simulink model "immd_eff1"  (R2013a)
settings: Solver=ode4  StartTime=0.0  StopTime=0.5  FixedStep=Ts  RelTol=1e-3
values from neighbouring files (symbols this model uses):
  Cdc = 200e-6    (= 0.0002)    [immd_design_elen.m]    (also in immd_efficiency.m = 5e-05; immd_simulation_base.m = 5e-05; sixth_harmonic_report.m = 0.003)
  fout = 50    [immd_base_varyingmod.m]    (also in immd_design_elen.m; immd_efficiency.m; immd_simulation_base.m)
  Lload = Xload/wout_fund    [acemp_sixth.m]    (also in immd_base_varyingmod.m = Xload/wout; immd_design_elen.m = Xload/wout; immd_efficiency.m = Xload/wout; immd_simulation_base.m = Xload/wout)
  ma = 1    [IMMD_design_tool_v01.m]    (also in IMMD_design_tool_v02.m = 0.9; immd_base_varyingmod.m; immd_design_elen.m = 0.8; immd_efficiency.m = 0.85)
  phase = zeros(1,max_number_module)    [immd_base_varyingmod.m]    (also in immd_design_elen.m = [0 0 0 0]; immd_simulation_base.m = zeros(1,n))
  R1 = 5    [immd_efficiency.m]    (also in immd_simulation_base.m)
  Rload = Zload*pf    [acemp_sixth.m]    (also in immd_base_varyingmod.m; immd_design_elen.m; immd_efficiency.m; immd_simulation_base.m)
  Ts = 1e-6    (= 1e-06)    [acemp_sixth.m]    (also in immd_base_varyingmod.m = 1e-05; immd_design_elen.m; immd_efficiency.m; immd_simulation_base.m)
  V1 = Vdc*(R1+Rrefl)/Rrefl    (= 526.262626263)    [immd_efficiency.m]    (also in immd_simulation_base.m = 425.252525253)
  wout = 2*pi*fout    (= 314.159265359)    [immd_base_varyingmod.m]    (also in immd_design_elen.m; immd_efficiency.m; immd_simulation_base.m)
libraries: powerlib x21, powerlib_meascontrol x7
settings Model: Creator=ugurm  LastModifiedBy=ugurm

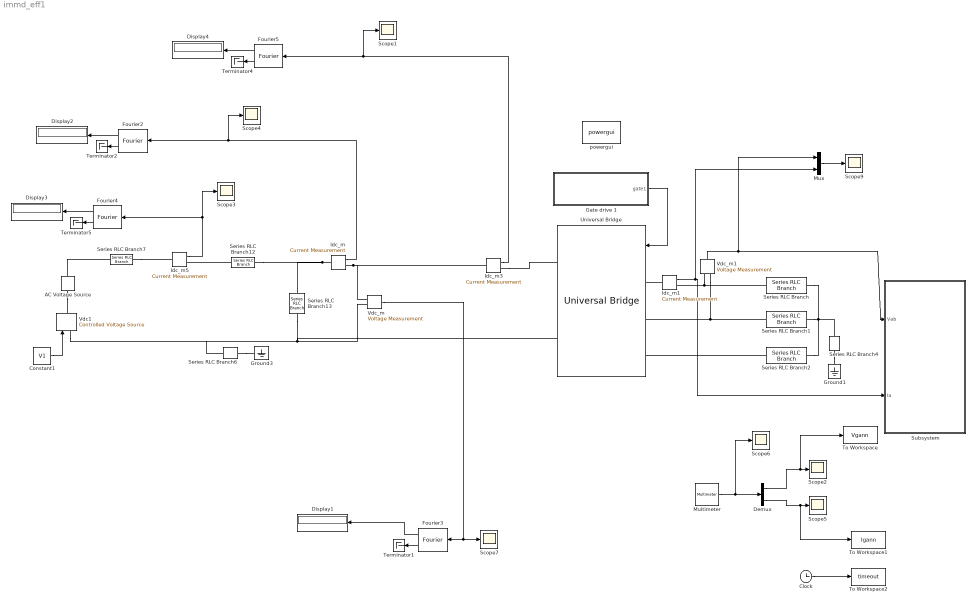
== system immd_eff1 ==
  AC Voltage Source : powerlib/Electrical Sources/AC Voltage Source  Amplitude=25  Phase=0  Frequency=6*fout  SampleTime=0  Measurements=None
  Clock : Clock
  Constant1 : Constant  Value=V1
  Demux : Demux  Outputs=2
  Display{1..4} (4 alike) : Display
  Fourier{2..5} (4 alike) : powerlib_meascontrol/Measurements/Fourier  Freq=fout  n=0  InInit=[0, 0]  Ts=Ts
  Gate drive 1 : Subsystem
  Ground1 : powerlib/Elements/Ground  LConnTagsString=a
  Ground3 : powerlib/Elements/Ground  LConnTagsString=a
  Idc_m{,1,3,5} (4 alike) : powerlib/Measurements/Current Measurement  PhasorSimulation=off  OutputType=Complex  PSBequivalent=0
  Multimeter : powerlib/Measurements/Multimeter  PhasorSimulation=off  OutputType=Complex  sel=[1 11]  L=16  Gain=[1 1]  yselected={'Usw1: Universal Bridge','Isw1: Universal Bridge'};  PSBOutputType=1  PSBequivalent=0  AxesSetting=[0,0.1,-100,100]  Display=0  SavedBlockNames=-11
  Mux : Mux  Inputs=2
  Scope{1..7,9} (8 alike) : Scope
      Scope1 settings: YMin=500  YMax=800  SaveName=idc1
      Scope2 settings: YMin=0  YMax=500
      Scope3 settings: YMin=24.9625  YMax=24.995  SaveName=ScopeData5
      Scope4 settings: YMin=500  YMax=800  SaveName=idc
      Scope5 settings: YMin=-450  YMax=450
      Scope6 settings: YMin=0  YMax=500  SaveName=ScopeData2
      Scope7 settings: YMin=150  YMax=550  SaveName=ScopeData7
      Scope9 settings: YMin=-450  YMax=450  SaveName=ScopeData6
  Series RLC Branch : powerlib/Elements/Series RLC Branch  LConnTagsString=__new0  RConnTagsString=__new0  BranchType=RL  Resistance=Rload  Inductance=Lload  SetiL0=off  InitialCurrent=0  Capacitance=1e-6  Setx0=off  InitialVoltage=0  Measurements=None
  Series RLC Branch1 : powerlib/Elements/Series RLC Branch  LConnTagsString=__new0  RConnTagsString=__new0  BranchType=RL  Resistance=Rload  Inductance=Lload  SetiL0=off  InitialCurrent=0  Capacitance=1e-6  Setx0=off  InitialVoltage=0  Measurements=None
  Series RLC Branch12 : powerlib/Elements/Series RLC Branch  LConnTagsString=__new0  RConnTagsString=__new0  BranchType=R  Resistance=R1  Inductance=Lload  SetiL0=off  InitialCurrent=0  Capacitance=1e-6  Setx0=off  InitialVoltage=0  Measurements=None
  Series RLC Branch13 : powerlib/Elements/Series RLC Branch  LConnTagsString=__new0  RConnTagsString=__new0  BranchType=C  Resistance=1e12  Inductance=Lload  SetiL0=off  InitialCurrent=0  Capacitance=Cdc  Setx0=off  InitialVoltage=0  Measurements=None
  Series RLC Branch2 : powerlib/Elements/Series RLC Branch  LConnTagsString=__new0  RConnTagsString=__new0  BranchType=RL  Resistance=Rload  Inductance=Lload  SetiL0=off  InitialCurrent=0  Capacitance=1e-6  Setx0=off  InitialVoltage=0  Measurements=None
  Series RLC Branch4 : powerlib/Elements/Series RLC Branch  LConnTagsString=__new0  RConnTagsString=__new0  BranchType=R  Resistance=1e12  Inductance=Lload  SetiL0=off  InitialCurrent=0  Capacitance=1e-6  Setx0=off  InitialVoltage=0  Measurements=None
  Series RLC Branch6 : powerlib/Elements/Series RLC Branch  LConnTagsString=__new0  RConnTagsString=__new0  BranchType=R  Resistance=1e12  Inductance=Lload  SetiL0=off  InitialCurrent=0  Capacitance=1e-6  Setx0=off  InitialVoltage=0  Measurements=None
  Series RLC Branch7 : powerlib/Elements/Series RLC Branch  LConnTagsString=__new0  RConnTagsString=__new0  BranchType=L  Resistance=1  Inductance=1000e-3  SetiL0=off  InitialCurrent=0  Capacitance=1e-6  Setx0=off  InitialVoltage=0  Measurements=None
  Subsystem : Subsystem
  Terminator{1..2,4..5} (4 alike) : Terminator
  To Workspace : ToWorkspace  VariableName=Vgann  SampleTime=-1
  To Workspace1 : ToWorkspace  VariableName=Igann  SampleTime=-1
  To Workspace2 : ToWorkspace  VariableName=timeout  SampleTime=-1
  Universal Bridge : powerlib/Power Electronics/Universal Bridge  Arms=3  SnubberResistance=1e5  SnubberCapacitance=inf  Device=IGBT / Diodes  Ron=1e-6  Lon=0  ForwardVoltages="[  0  0  ]"  ForwardVoltage=0  GTOparameters=[ 10e-6 , 20e-6 ]  IGBTparameters=[0,0]  Measurements=All voltages and currents  Measurements_2=None  converterType=Rectifier
  Vdc1 : powerlib/Electrical Sources/Controlled Voltage Source  Initialize=off  Source_Type=DC  Amplitude=200  Phase=0  Frequency=0  Measurements=None
  Vdc_m : powerlib/Measurements/Voltage Measurement  PhasorSimulation=off  OutputType=Complex  PSBequivalent=0
  Vdc_m1 : powerlib/Measurements/Voltage Measurement  PhasorSimulation=off  OutputType=Complex  PSBequivalent=0
  powergui : powerlib/powergui  Priority=1  SimulationMode=Discrete  SolverType=Tustin  SampleTime=Ts  frequency=60  SPID=off  DisableSnubberDevices=off  DisableRonSwitches=off  DisableVfSwitches=off  SwTol=0  Interpol=off  DisplayEquations=off  frequencyindice=0  Pbase=100e6  ErrMax=1e-4  Iterations=50  UnitsV=kV  UnitsW=MW  FunctionMessages=off  echomessages=off  HookPort=off  EnableUseOfTLC=off  x0status=blocks  RestoreLinks=warning  ResistiveCurrentMeasurement=off  Frange=[0:2:500]  Ylog=off  Xlog=on  ShowGrid=off  save=off  variable=ZData  structure=idc3  ZoomFFT=off  StartTime=0.02  cycles=3  DisplayStyle=1  fundamental=50  FreqAxis=off  MaxFrequency=10000  frequencyindicesteady=1  RmsSteady=1  display=off  Ts=0  methode=off
  wires:
  Gate drive 1/1(gate1) -> Universal Bridge/1
  Vdc_m1/1 -> Mux/1, Subsystem/1(Vab)
  Idc_m1/1 -> Mux/2, Subsystem/2(Ia)
  Idc_m/1 -> Scope4/1, Fourier2/1
  Constant1/1 -> Vdc1/1
  Fourier2/1 -> Display2/1
  Fourier2/2 -> Terminator2/1
  Idc_m5/1 -> Scope3/1, Fourier4/1
  Fourier4/1 -> Display3/1
  Fourier4/2 -> Terminator5/1
  Fourier3/1 -> Display1/1
  Fourier3/2 -> Terminator1/1
  Vdc_m/1 -> Fourier3/1, Scope7/1
  Mux/1 -> Scope9/1
  Idc_m3/1 -> Scope1/1, Fourier5/1
  Fourier5/1 -> Display4/1
  Fourier5/2 -> Terminator4/1
  Multimeter/1 -> Scope6/1, Demux/1
  Demux/1 -> To Workspace/1, Scope2/1
  Demux/2 -> To Workspace1/1, Scope5/1
  Clock/1 -> To Workspace2/1
  connections:
  Idc_m/RConn1 -- Idc_m3/LConn1 -- Vdc_m/LConn1
  Idc_m1/LConn1 -- Universal Bridge/LConn1
  Series RLC Branch1/LConn1 -- Universal Bridge/LConn2 -- Vdc_m1/LConn2
  Series RLC Branch2/LConn1 -- Universal Bridge/LConn3
  Series RLC Branch/LConn1 -- Idc_m1/RConn1 -- Vdc_m1/LConn1
  Series RLC Branch/RConn1 -- Series RLC Branch2/RConn1 -- Series RLC Branch4/LConn1 -- Series RLC Branch1/RConn1
  Series RLC Branch4/RConn1 -- Ground1/LConn1
  Series RLC Branch13/RConn1 -- Vdc_m/LConn2 -- Universal Bridge/RConn2 -- Vdc1/LConn1 -- Series RLC Branch6/LConn1
  Series RLC Branch6/RConn1 -- Ground3/LConn1
  Idc_m/LConn1 -- Series RLC Branch12/LConn1 -- Series RLC Branch13/LConn1
  Series RLC Branch12/RConn1 -- Idc_m5/RConn1
  Series RLC Branch7/LConn1 -- Idc_m5/LConn1
  AC Voltage Source/LConn1 -- Vdc1/RConn1
  Series RLC Branch7/RConn1 -- AC Voltage Source/RConn1
  Idc_m3/RConn1 -- Universal Bridge/RConn1

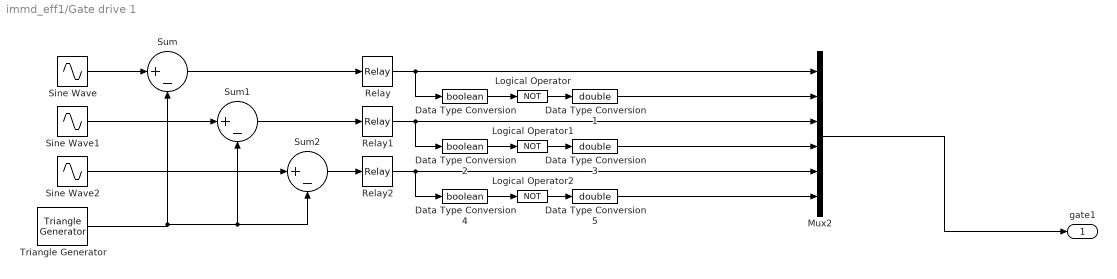
== system immd_eff1/Gate drive 1 ==
  Data Type Conversion : DataTypeConversion  OutDataTypeStr=boolean
  Data Type Conversion1 : DataTypeConversion  OutDataTypeStr=double
  Data Type Conversion2 : DataTypeConversion  OutDataTypeStr=boolean
  Data Type Conversion3 : DataTypeConversion  OutDataTypeStr=double
  Data Type Conversion4 : DataTypeConversion  OutDataTypeStr=boolean
  Data Type Conversion5 : DataTypeConversion  OutDataTypeStr=double
  Logical Operator : Logic  Operator=NOT  AllPortsSameDT=off  OutDataTypeStr=boolean
  Logical Operator1 : Logic  Operator=NOT  AllPortsSameDT=off  OutDataTypeStr=boolean
  Logical Operator2 : Logic  Operator=NOT  AllPortsSameDT=off  OutDataTypeStr=boolean
  Mux2 : Mux  Inputs=6
  Relay : Relay
  Relay1 : Relay
  Relay2 : Relay
  Sine Wave : Sin  Amplitude=ma  Frequency=wout  SampleTime=0
  Sine Wave1 : Sin  Amplitude=ma  Frequency=wout  Phase=-2*pi/3  SampleTime=0
  Sine Wave2 : Sin  Amplitude=ma  Frequency=wout  Phase=2*pi/3  SampleTime=0
  Sum : Sum  Inputs=|+-
  Sum1 : Sum  Inputs=|+-
  Sum2 : Sum  Inputs=|+-
  Triangle Generator : powerlib_meascontrol/Pulse & Signal Generators/Triangle Generator  Freq=fsw  Phase=phase(1)  Ts=Ts
  gate1 : Outport
  wires:
  Sine Wave/1 -> Sum/1
  Triangle Generator/1 -> Sum1/2, Sum2/2, Sum/2
  Sine Wave1/1 -> Sum1/1
  Sine Wave2/1 -> Sum2/1
  Sum/1 -> Relay/1
  Sum1/1 -> Relay1/1
  Sum2/1 -> Relay2/1
  Data Type Conversion/1 -> Logical Operator/1
  Relay/1 -> Data Type Conversion/1, Mux2/1
  Logical Operator/1 -> Data Type Conversion1/1
  Data Type Conversion1/1 -> Mux2/2
  Data Type Conversion2/1 -> Logical Operator1/1
  Relay1/1 -> Data Type Conversion2/1, Mux2/3
  Logical Operator1/1 -> Data Type Conversion3/1
  Data Type Conversion3/1 -> Mux2/4
  Data Type Conversion4/1 -> Logical Operator2/1
  Relay2/1 -> Data Type Conversion4/1, Mux2/5
  Logical Operator2/1 -> Data Type Conversion5/1
  Data Type Conversion5/1 -> Mux2/6
  Mux2/1 -> gate1/1

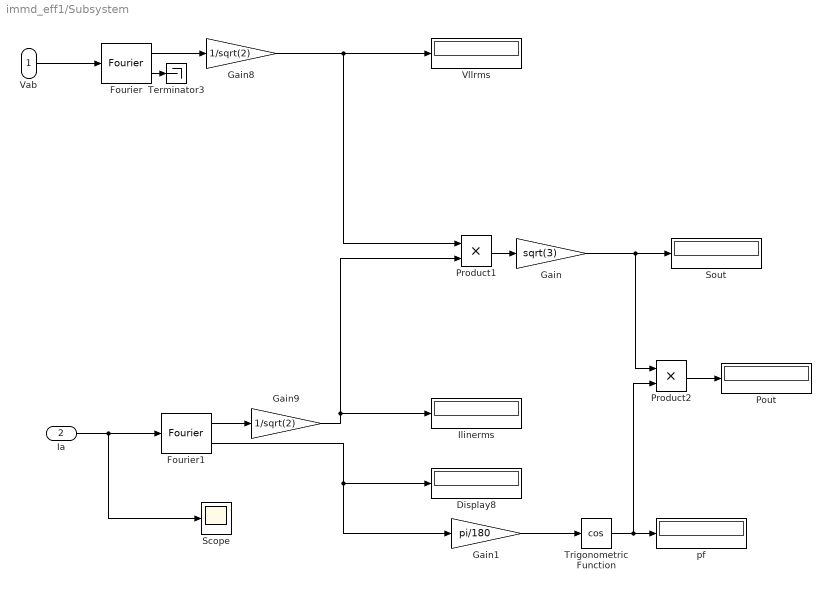
== system immd_eff1/Subsystem ==
  Vab : Inport
  Ia : Inport  Port=2
  Display8 : Display
  Fourier : powerlib_meascontrol/Measurements/Fourier  Freq=fout  n=1  InInit=[0, 0]  Ts=Ts
  Fourier1 : powerlib_meascontrol/Measurements/Fourier  Freq=fout  n=1  InInit=[0, 0]  Ts=Ts
  Gain : Gain  Gain=sqrt(3)
  Gain1 : Gain  Gain=pi/180
  Gain8 : Gain  Gain=1/sqrt(2)
  Gain9 : Gain  Gain=1/sqrt(2)
  "Ilinerms " : Display
  Pout : Display
  Product1 : Product
  Product2 : Product
  Scope : Scope
      settings: YMin=-10  YMax=10  SaveName=ScopeData4
  Sout : Display
      settings: Format=short_e
  Terminator3 : Terminator
  Trigonometric Function : Trigonometry  Operator=cos
  "Vllrms " : Display
  pf : Display
  wires:
  Gain8/1 -> Product1/1, "Vllrms "/1
  Gain9/1 -> "Ilinerms "/1, Product1/2
  Ia/1 -> Scope/1, Fourier1/1
  Fourier1/1 -> Gain9/1
  Vab/1 -> Fourier/1
  Fourier/1 -> Gain8/1
  Product1/1 -> Gain/1
  Gain/1 -> Product2/1, Sout/1
  Fourier1/2 -> Gain1/1, Display8/1
  Trigonometric Function/1 -> Product2/2, pf/1
  Gain1/1 -> Trigonometric Function/1
  Product2/1 -> Pout/1
  Fourier/2 -> Terminator3/1
